simulink model "Rasmusson"  (Simulink 7.1)
settings: Solver=ode15s  StartTime=0.0  StopTime=500  FixedStep=1e-4  MaxStep=0.1  RelTol=1e-6
values from neighbouring files (symbols this model uses):
  Acap = 1.534e-4    (= 0.0001534)    [MMparameters.m]
  aKss = 0.417069e-3    (= 0.000417069)    [MMparameters.m]
  ato_f = 0.265563e-2    (= 0.00265563)    [MMparameters.m]
  ato_s = 0.417069e-3    (= 0.000417069)    [MMparameters.m]
  aur = 0.417069e-3    (= 0.000417069)    [MMparameters.m]
  C2 = 0.124216e-3    (= 0.000124216)    [MMparameters.m]
  C3 = 0.578679e-8    (= 5.78679e-09)    [MMparameters.m]
  C4 = 0.119816e-12    (= 1.19816e-13)    [MMparameters.m]
  Cai = 0.115001    [MMparameters.m]
  CaJSR = 1299.50    (= 1299.5)    [MMparameters.m]
  CaNSR = 1299.50    (= 1299.5)    [MMparameters.m]
  Cao = 1800    [MMparameters.m]
  Cass = 0.115001    [MMparameters.m]
  CK1 = 0.992513e-3    (= 0.000992513)    [MMparameters.m]
  CK2 = 0.641229e-3    (= 0.000641229)    [MMparameters.m]
  Cm = 1.0    (= 1)    [MMparameters.m]
  CMDN_tot = 50.0    (= 50)    [MMparameters.m]
  CNa1 = 0.279132e-3    (= 0.000279132)    [MMparameters.m]
  CNa2 = 0.020752    [MMparameters.m]
  CSQN_tot = 15000.0    (= 15000)    [MMparameters.m]
  ECa_L = 63.0    (= 63)    [MMparameters.m]
  ECl = -40.0    (= -40)    [MMparameters.m]
  F = 96.5    [MMparameters.m]
  GCab = 0.000367    [MMparameters.m]
  GCaL = 0.1729    [MMparameters.m]
  GCl_Ca = 10.0    (= 10)    [MMparameters.m]
  GKr = 0.078    [MMparameters.m]
  GKs = 0.00575    [MMparameters.m]
  GKss = 0.050    (= 0.05)    [MMparameters.m]
  GKtof = 0.4067    [MMparameters.m]
  GKtos = 0.0    (= 0)    [MMparameters.m]
  GKur = 0.160    (= 0.16)    [MMparameters.m]
  GNa = 13.0    (= 13)    [MMparameters.m]
  GNab = 0.0026    [MMparameters.m]
  HTRPN_tot = 140.0    (= 140)    [MMparameters.m]
  HTRPNCa = 125.290    (= 125.29)    [MMparameters.m]
  I1 = 0.497923e-18    (= 4.97923e-19)    [MMparameters.m]
  I1Na = 0.673345e-6    (= 6.73345e-07)    [MMparameters.m]
  I2 = 0.345847e-13    (= 3.45847e-14)    [MMparameters.m]
  I2Na = 0.155787e-8    (= 1.55787e-09)    [MMparameters.m]
  I3 = 0.185106e-13    (= 1.85106e-14)    [MMparameters.m]
  ICaL_max = 7.0    (= 7)    [MMparameters.m]
  ICNa2 = 0.0113879    [MMparameters.m]
  ICNa3 = 0.342780    (= 0.34278)    [MMparameters.m]
  IFNa = 0.153176e-3    (= 0.000153176)    [MMparameters.m]
  IK = 0.319129e-4    (= 3.19129e-05)    [MMparameters.m]
  iKss = 1.0    (= 1)    [MMparameters.m]
  INaK_max = 0.88    [MMparameters.m]
  Ip_Ca_max = 1.0    (= 1)    [MMparameters.m]
  ito_f = 0.999977    [MMparameters.m]
  ito_s = 0.998543    [MMparameters.m]
  iur = 0.998543    [MMparameters.m]
  ka1 = 0.006075    [MMparameters.m]
  ka2 = 0.07125    [MMparameters.m]
  kb = 0.036778    [MMparameters.m]
  kb1 = 0.00405    [MMparameters.m]
  kb2 = 0.965    [MMparameters.m]
  kc1 = 0.009    [MMparameters.m]
  kc2 = 0.0008    [MMparameters.m]
  kf = 0.023761    [MMparameters.m]
  khtrpn1 = 0.00237    [MMparameters.m]
  khtrpn2 = 3.2e-5    (= 3.2e-05)    [MMparameters.m]
  Ki = 143720    [MMparameters.m]
  kltrpn1 = 0.0327    [MMparameters.m]
  kltrpn2 = 0.0196    [MMparameters.m]
  Km_Ca = 1380    [MMparameters.m]
  Km_Cl = 10.0    (= 10)    [MMparameters.m]
  Km_CMDN = 0.238    [MMparameters.m]
  Km_CSQN = 800.0    (= 800)    [MMparameters.m]
  Km_Ko = 1500    [MMparameters.m]
  Km_Na = 87500    [MMparameters.m]
  Km_Nai = 21000    [MMparameters.m]
  Km_p_Ca = 0.5    [MMparameters.m]
  Km_up = 0.5    [MMparameters.m]
  kNaCa = 292.8    [MMparameters.m]
  Ko = 5400    [MMparameters.m]
  Kpc_half = 20.0    (= 20)    [MMparameters.m]
  Kpc_max = 0.23324    [MMparameters.m]
  Kpcb = 0.0005    [MMparameters.m]
  ksat = 0.1    [MMparameters.m]
  LTRPN_tot = 70.0    (= 70)    [MMparameters.m]
  LTRPNCa = 11.2684    [MMparameters.m]
  Nai = 14237.1    [MMparameters.m]
  Nao = 140000    [MMparameters.m]
  nKs = 0.262753e-3    (= 0.000262753)    [MMparameters.m]
  nu1 = 4.5    [MMparameters.m]
  nu2 = 1.74e-5    (= 1.74e-05)    [MMparameters.m]
  nu3 = 0.45    [MMparameters.m]
  O = 0.930308e-18    (= 9.30308e-19)    [MMparameters.m]
  OK = 0.175298e-3    (= 0.000175298)    [MMparameters.m]
  ONa = 0.713483e-6    (= 7.13483e-07)    [MMparameters.m]
  PC2 = 0.167740e-3    (= 0.00016774)    [MMparameters.m]
  PO1 = 0.149102e-4    (= 1.49102e-05)    [MMparameters.m]
  PO2 = 0.951726e-10    (= 9.51726e-11)    [MMparameters.m]
  PRyR = 0.0    (= 0)    [MMparameters.m]
  R = 8.314    [MMparameters.m]
  T = 298    [MMparameters.m]
  tautr = 20.0    (= 20)    [MMparameters.m]
  tauxfer = 8.0    (= 8)    [MMparameters.m]
  V = -82.4202    [MMparameters.m]
  VJSR = 0.12e-6    (= 1.2e-07)    [MMparameters.m]
  Vmyo = 25.84e-6    (= 2.584e-05)    [MMparameters.m]
  VNSR = 2.098e-6    (= 2.098e-06)    [MMparameters.m]
  Vss = 1.485e-9    (= 1.485e-09)    [MMparameters.m]
  yita = 0.35    [MMparameters.m]
(part 1 of 2)
settings Model: Creator=yunchen  LastModifiedBy=yunchen  BufferReuse=off
settings SolverCC: MaxOrder=2
settings DataIOCC: LimitDataPoints=off  SaveFinalState=on  SaveOutput=off  SignalLoggingName=sigsOut
settings OptimizationCC: InlineParams=on  OptimizeBlockIOStorage=off  BufferReuse=off  ExpressionFolding=off  LocalBlockOutputs=off
settings DebuggingCC: SaveWithParameterizedLinksMsg=none  MultiTaskDSMMsg=warning  MultiTaskCondExecSysMsg=none  CheckMatrixSingularityMsg=warning

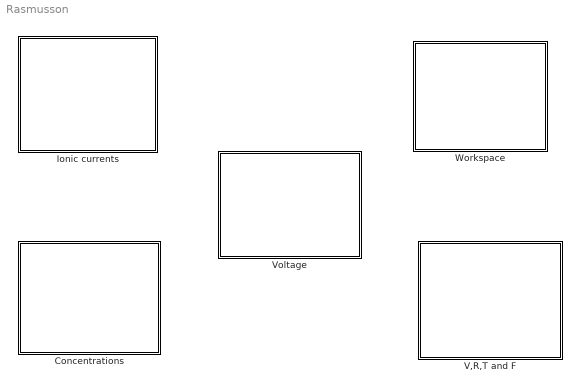
== system Rasmusson ==
  Concentrations : Subsystem
  Ionic currents : Subsystem
  V,R,T and F : Subsystem
  Voltage : Subsystem
  Workspace : Subsystem

== system Rasmusson/Concentrations ==
  ACdivideVF : Subsystem
  Caconcentration : Subsystem
  Ki : Subsystem
  Nai : Subsystem

== system Rasmusson/Ionic currents ==
  EK : Subsystem
  ENa : Subsystem
  ICaL : Subsystem
  ICab : Subsystem
  IK1 : Subsystem
  IKr : Subsystem
  IKs : Subsystem
  IKss : Subsystem
  IKto,f : Subsystem
  IKto,s : Subsystem
  IKur : Subsystem
  INa : Subsystem
  INaCa : Subsystem
  INaK : Subsystem
  INab : Subsystem
  IpCa : Subsystem

== system Rasmusson/V,R,T and F ==
  Divide : Product  Inputs=*/  OutDataType=sfix(16)  OutScaling=2^-10
  Divide1 : Product  Inputs=*/  OutDataType=sfix(16)  OutScaling=2^-10
  F : Constant  Value=F  OutDataType=sfix(16)  OutScaling=2^0
  Product : Product  OutDataType=sfix(16)  OutScaling=2^0  RndMeth=Zero
  R : Constant  Value=R  OutDataType=sfix(16)  OutScaling=2^0
  T : Constant  Value=T  OutDataType=sfix(16)  OutScaling=2^0
  tag scope: RTdivideF=global, VFdivideRT=global
  wires:
  R/1 -> Product/1
  T/1 -> Product/2
  Product/1 -> Divide/1
  F/1 -> Divide/2
  Divide/1 -> [RTdivideF], Divide1/2
  [volt] -> Divide1/1
  Divide1/1 -> [VFdivideRT]

== system Rasmusson/Voltage ==
  Cacurrents : Subsystem
  ICaCl : Subsystem
  Kdynamics : Subsystem
  Nadynamics : Subsystem
  Voltage : Subsystem

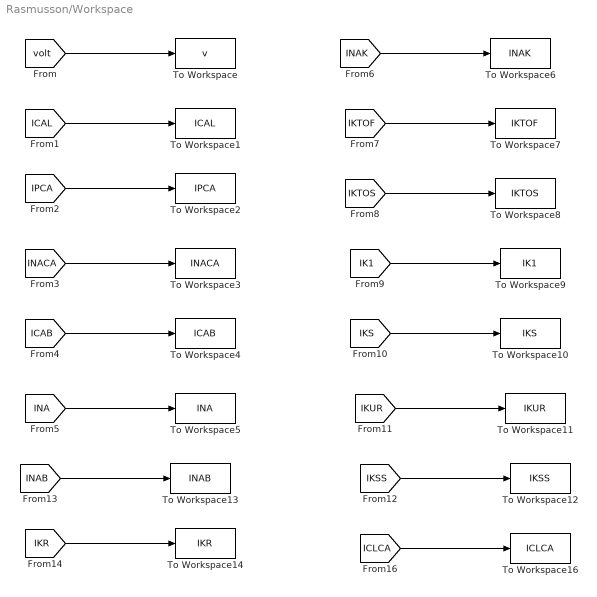
== system Rasmusson/Workspace ==
  To Workspace : ToWorkspace  VariableName=v  SampleTime=-1  SaveFormat=Array
  To Workspace1 : ToWorkspace  VariableName=ICAL  SampleTime=-1  SaveFormat=Array
  To Workspace10 : ToWorkspace  VariableName=IKS  SampleTime=-1  SaveFormat=Array
  To Workspace11 : ToWorkspace  VariableName=IKUR  SampleTime=-1  SaveFormat=Array
  To Workspace12 : ToWorkspace  VariableName=IKSS  SampleTime=-1  SaveFormat=Array
  To Workspace13 : ToWorkspace  VariableName=INAB  SampleTime=-1  SaveFormat=Array
  To Workspace14 : ToWorkspace  VariableName=IKR  SampleTime=-1  SaveFormat=Array
  To Workspace16 : ToWorkspace  VariableName=ICLCA  SampleTime=-1  SaveFormat=Array
  To Workspace2 : ToWorkspace  VariableName=IPCA  SampleTime=-1  SaveFormat=Array
  To Workspace3 : ToWorkspace  VariableName=INACA  SampleTime=-1  SaveFormat=Array
  To Workspace4 : ToWorkspace  VariableName=ICAB  SampleTime=-1  SaveFormat=Array
  To Workspace5 : ToWorkspace  VariableName=INA  SampleTime=-1  SaveFormat=Array
  To Workspace6 : ToWorkspace  VariableName=INAK  SampleTime=-1  SaveFormat=Array
  To Workspace7 : ToWorkspace  VariableName=IKTOF  SampleTime=-1  SaveFormat=Array
  To Workspace8 : ToWorkspace  VariableName=IKTOS  SampleTime=-1  SaveFormat=Array
  To Workspace9 : ToWorkspace  VariableName=IK1  SampleTime=-1  SaveFormat=Array
  wires:
  [volt] -> To Workspace/1
  [ICAL] -> To Workspace1/1
  [IPCA] -> To Workspace2/1
  [INACA] -> To Workspace3/1
  [ICAB] -> To Workspace4/1
  [INA] -> To Workspace5/1
  [INAK] -> To Workspace6/1
  [IKTOF] -> To Workspace7/1
  [IKTOS] -> To Workspace8/1
  [IK1] -> To Workspace9/1
  [IKS] -> To Workspace10/1
  [IKUR] -> To Workspace11/1
  [IKSS] -> To Workspace12/1
  [INAB] -> To Workspace13/1
  [IKR] -> To Workspace14/1
  [ICLCA] -> To Workspace16/1

== system Rasmusson/Concentrations/ACdivideVF ==
  Acap : Constant  Value=Acap  OutDataType=sfix(16)  OutScaling=2^0
  Cm : Constant  Value=Cm  OutDataType=sfix(16)  OutScaling=2^0
  Divide : Product  Inputs=**//  OutDataType=sfix(16)  OutScaling=2^-10
  F : Constant  Value=F  OutDataType=sfix(16)  OutScaling=2^0
  Vmyo : Constant  Value=Vmyo  OutDataType=sfix(16)  OutScaling=2^0
  tag scope: ACdivideVF=global
  wires:
  Acap/1 -> Divide/1
  Cm/1 -> Divide/2
  Vmyo/1 -> Divide/3
  F/1 -> Divide/4
  Divide/1 -> [ACdivideVF]

== system Rasmusson/Concentrations/Caconcentration ==
  Cabuffering : Subsystem
  Caconcentration : Subsystem
  Cafluxes : Subsystem
  Ryanodine_receptors : Subsystem

== system Rasmusson/Concentrations/Ki ==
  Add : Sum  Inputs=++++++++  OutDataType=sfix(16)  OutScaling=2^-10
  Gain : Gain  Gain=-1  ParameterDataType=sfix(16)  ParameterScaling=2^0  OutDataType=sfix(16)  OutScaling=2^0
  Gain1 : Gain  Gain=-2  ParameterDataType=sfix(16)  ParameterScaling=2^0  OutDataType=sfix(16)  OutScaling=2^0
  Integrator : Integrator  InitialConditionSource=external  InitialCondition=143720
  Ki : Constant  Value=Ki  OutDataType=sfix(16)  OutScaling=2^0
  Product : Product  OutDataType=sfix(16)  OutScaling=2^0  RndMeth=Zero
  tag scope: Ki=global
  wires:
  Integrator/1 -> [Ki]
  Gain/1 -> Integrator/1
  Product/1 -> Gain/1
  Add/1 -> Product/2
  [IKTOS] -> Add/2
  [IKTOF] -> Add/1
  [IK1] -> Add/3
  [IKS] -> Add/4
  [ACdivideVF] -> Product/1
  [IKSS] -> Add/5
  [IKUR] -> Add/6
  [IKR] -> Add/7
  Gain1/1 -> Add/8
  [INAK] -> Gain1/1
  Ki/1 -> Integrator/2

== system Rasmusson/Concentrations/Nai ==
  Add : Sum  Inputs=++++  OutDataType=sfix(16)  OutScaling=2^-10
  Gain : Gain  Gain=-1  ParameterDataType=sfix(16)  ParameterScaling=2^0  OutDataType=sfix(16)  OutScaling=2^0
  Gain1 : Gain  Gain=3  ParameterDataType=sfix(16)  ParameterScaling=2^0  OutDataType=sfix(16)  OutScaling=2^0
  Gain2 : Gain  Gain=3  ParameterDataType=sfix(16)  ParameterScaling=2^0  OutDataType=sfix(16)  OutScaling=2^0
  Integrator : Integrator  InitialConditionSource=external  InitialCondition=14237.1
  Nai : Constant  Value=Nai  OutDataType=sfix(16)  OutScaling=2^0
  Product : Product  OutDataType=sfix(16)  OutScaling=2^0  RndMeth=Zero
  tag scope: Nai=global
  wires:
  Integrator/1 -> [Nai]
  Gain/1 -> Integrator/1
  Product/1 -> Gain/1
  Add/1 -> Product/2
  Gain1/1 -> Add/4
  Gain2/1 -> Add/3
  [INAB] -> Add/2
  [INA] -> Add/1
  [INACA] -> Gain2/1
  [INAK] -> Gain1/1
  [ACdivideVF] -> Product/1
  Nai/1 -> Integrator/2

== system Rasmusson/Ionic currents/EK ==
  Divide : Product  Inputs=*/  OutDataType=sfix(16)  OutScaling=2^-10
  Ko : Constant  Value=Ko  OutDataType=sfix(16)  OutScaling=2^0
  Math Function : Math  Operator=log  OutDataType=sfix(16)  OutScaling=2^0  SaturateOnIntegerOverflow=on
  Product : Product  OutDataType=sfix(16)  OutScaling=2^0  RndMeth=Zero
  tag scope: EK=global
  wires:
  Ko/1 -> Divide/1
  [Ki] -> Divide/2
  Divide/1 -> Math Function/1
  Product/1 -> [EK]
  Math Function/1 -> Product/2
  [RTdivideF] -> Product/1

== system Rasmusson/Ionic currents/ENa ==
  Add : Sum  OutDataType=sfix(16)  OutScaling=2^-10
  Add1 : Sum  OutDataType=sfix(16)  OutScaling=2^-10
  Divide : Product  Inputs=*/  OutDataType=sfix(16)  OutScaling=2^-10
  Divide1 : Product  Inputs=**  OutDataType=sfix(16)  OutScaling=2^-10
  Gain : Gain  Gain=0.9  ParameterDataType=sfix(16)  ParameterScaling=2^0  OutDataType=sfix(16)  OutScaling=2^0
  Gain1 : Gain  Gain=0.1  ParameterDataType=sfix(16)  ParameterScaling=2^0  OutDataType=sfix(16)  OutScaling=2^0
  Gain2 : Gain  Gain=0.9  ParameterDataType=sfix(16)  ParameterScaling=2^0  OutDataType=sfix(16)  OutScaling=2^0
  Gain3 : Gain  Gain=0.1  ParameterDataType=sfix(16)  ParameterScaling=2^0  OutDataType=sfix(16)  OutScaling=2^0
  Ko : Constant  Value=Ko  OutDataType=sfix(16)  OutScaling=2^0
  Math Function : Math  Operator=log  OutDataType=sfix(16)  OutScaling=2^0  SaturateOnIntegerOverflow=on
  Nao : Constant  Value=Nao  OutDataType=sfix(16)  OutScaling=2^0
  tag scope: ENa=global
  wires:
  Divide/1 -> Math Function/1
  Gain/1 -> Add/1
  Add/1 -> Divide/1
  Gain1/1 -> Add/2
  Add1/1 -> Divide/2
  Gain2/1 -> Add1/1
  Gain3/1 -> Add1/2
  Math Function/1 -> Divide1/1
  [RTdivideF] -> Divide1/2
  Divide1/1 -> [ENa]
  [Ki] -> Gain3/1
  [Nai] -> Gain2/1
  Nao/1 -> Gain/1
  Ko/1 -> Gain1/1

== system Rasmusson/Ionic currents/ICaL ==
  ECaL : Constant  Value=ECa_L  OutDataType=sfix(16)  OutScaling=2^0
  GCaL : Constant  Value=GCaL  OutDataType=sfix(16)  OutScaling=2^0
  O : Subsystem
  Product : Product  Inputs=3  OutDataType=sfix(16)  OutScaling=2^0  RndMeth=Zero
  Subtract : Sum  Inputs=+-  OutDataType=sfix(16)  OutScaling=2^-10
  tag scope: ICAL=global
  wires:
  Product/1 -> [ICAL]
  [O] -> Product/2
  Subtract/1 -> Product/3
  [volt] -> Subtract/1
  GCaL/1 -> Product/1
  ECaL/1 -> Subtract/2

== system Rasmusson/Ionic currents/ICab ==
  ECaN : Subsystem
  GCab : Constant  Value=GCab  OutDataType=sfix(16)  OutScaling=2^0
  Product : Product  OutDataType=sfix(16)  OutScaling=2^0  RndMeth=Zero
  Subtract : Sum  Inputs=+-  OutDataType=sfix(16)  OutScaling=2^-10
  tag scope: ICAB=global
  wires:
  Product/1 -> [ICAB]
  [volt] -> Subtract/1
  [ECaN] -> Subtract/2
  Subtract/1 -> Product/2
  GCab/1 -> Product/1

== system Rasmusson/Ionic currents/IK1 ==
  Add : Sum  OutDataType=sfix(16)  OutScaling=2^-10
  Add1 : Sum  OutDataType=sfix(16)  OutScaling=2^-10
  Constant1 : Constant  Value=210  OutDataType=sfix(16)  OutScaling=2^0
  Constant2 : Constant  OutDataType=sfix(16)  OutScaling=2^0
  Divide : Product  Inputs=*/  OutDataType=sfix(16)  OutScaling=2^-10
  Divide1 : Product  Inputs=*/  OutDataType=sfix(16)  OutScaling=2^-10
  Gain : Gain  Gain=0.2938  ParameterDataType=sfix(16)  ParameterScaling=2^0  OutDataType=sfix(16)  OutScaling=2^0
  Gain1 : Gain  Gain=0.0896  ParameterDataType=sfix(16)  ParameterScaling=2^0  OutDataType=sfix(16)  OutScaling=2^0
  Ko : Constant  Value=Ko  OutDataType=sfix(16)  OutScaling=2^0
  Math Function : Math  OutDataType=sfix(16)  OutScaling=2^0  SaturateOnIntegerOverflow=on
  Product : Product  OutDataType=sfix(16)  OutScaling=2^0  RndMeth=Zero
  Subtract : Sum  Inputs=+-  OutDataType=sfix(16)  OutScaling=2^-10
  tag scope: IK1=global
  wires:
  Product/1 -> Gain/1
  Gain/1 -> [IK1]
  Divide/1 -> Product/1
  Ko/1 -> Divide/1, Add/1
  Add/1 -> Divide/2
  Constant1/1 -> Add/2
  [volt] -> Subtract/1
  [EK] -> Subtract/2
  Divide1/1 -> Product/2
  Subtract/1 -> Divide1/1, Gain1/1
  Add1/1 -> Divide1/2
  Constant2/1 -> Add1/2
  Math Function/1 -> Add1/1
  Gain1/1 -> Math Function/1

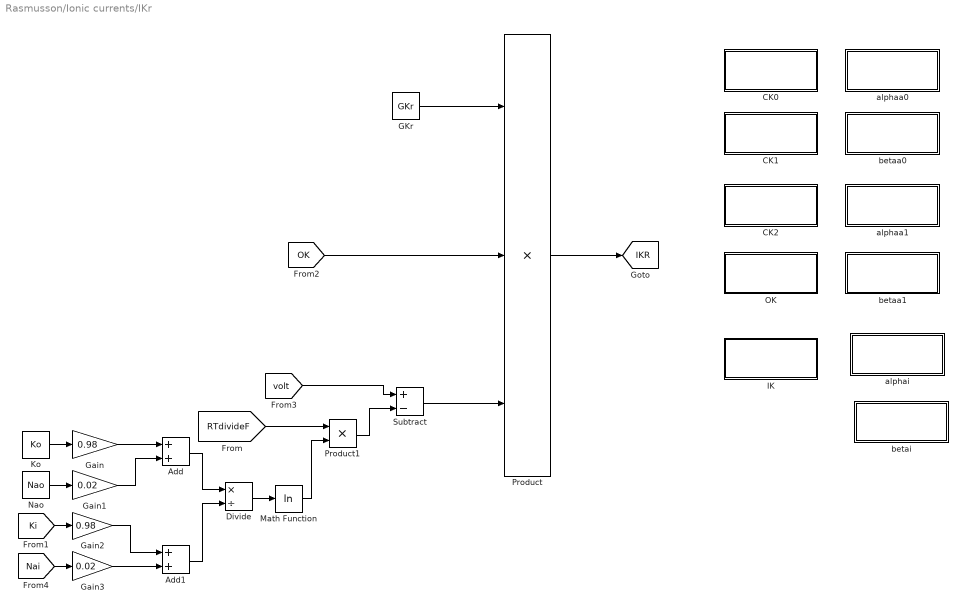
== system Rasmusson/Ionic currents/IKr ==
  Add : Sum  OutDataType=sfix(16)  OutScaling=2^-10
  Add1 : Sum  OutDataType=sfix(16)  OutScaling=2^-10
  CK0 : Subsystem
  CK1 : Subsystem
  CK2 : Subsystem
  Divide : Product  Inputs=*/  OutDataType=sfix(16)  OutScaling=2^-10
  GKr : Constant  Value=GKr  OutDataType=sfix(16)  OutScaling=2^0
  Gain : Gain  Gain=0.98  ParameterDataType=sfix(16)  ParameterScaling=2^0  OutDataType=sfix(16)  OutScaling=2^0
  Gain1 : Gain  Gain=0.02  ParameterDataType=sfix(16)  ParameterScaling=2^0  OutDataType=sfix(16)  OutScaling=2^0
  Gain2 : Gain  Gain=0.98  ParameterDataType=sfix(16)  ParameterScaling=2^0  OutDataType=sfix(16)  OutScaling=2^0
  Gain3 : Gain  Gain=0.02  ParameterDataType=sfix(16)  ParameterScaling=2^0  OutDataType=sfix(16)  OutScaling=2^0
  IK : Subsystem
  Ko : Constant  Value=Ko  OutDataType=sfix(16)  OutScaling=2^0
  Math Function : Math  Operator=log  OutDataType=sfix(16)  OutScaling=2^0  SaturateOnIntegerOverflow=on
  Nao : Constant  Value=Nao  OutDataType=sfix(16)  OutScaling=2^0
  OK : Subsystem
  Product : Product  Inputs=3  OutDataType=sfix(16)  OutScaling=2^0  RndMeth=Zero
  Product1 : Product  OutDataType=sfix(16)  OutScaling=2^0  RndMeth=Zero
  Subtract : Sum  Inputs=+-  OutDataType=sfix(16)  OutScaling=2^-10
  alphaa0 : Subsystem
  alphaa1 : Subsystem
  alphai : Subsystem
  betaa0 : Subsystem
  betaa1 : Subsystem
  betai : Subsystem
  tag scope: IKR=global
  wires:
  Product/1 -> [IKR]
  GKr/1 -> Product/1
  [OK] -> Product/2
  Subtract/1 -> Product/3
  [volt] -> Subtract/1
  Product1/1 -> Subtract/2
  [RTdivideF] -> Product1/1
  Math Function/1 -> Product1/2
  Divide/1 -> Math Function/1
  Add/1 -> Divide/1
  Add1/1 -> Divide/2
  Gain/1 -> Add/1
  Ko/1 -> Gain/1
  Gain1/1 -> Add/2
  Nao/1 -> Gain1/1
  [Ki] -> Gain2/1
  [Nai] -> Gain3/1
  Gain2/1 -> Add1/1
  Gain3/1 -> Add1/2

== system Rasmusson/Ionic currents/IKs ==
  Divide : Product  Inputs=***  OutDataType=sfix(16)  OutScaling=2^-10
  GKs : Constant  Value=GKs  OutDataType=sfix(16)  OutScaling=2^0
  Product : Product  OutDataType=sfix(16)  OutScaling=2^0  RndMeth=Zero
  Subtract : Sum  Inputs=+-  OutDataType=sfix(16)  OutScaling=2^-10
  alphan : Subsystem
  betan : Subsystem
  nKs : Subsystem
  tag scope: IKS=global
  wires:
  GKs/1 -> Divide/1
  Product/1 -> Divide/2
  Subtract/1 -> Divide/3
  Divide/1 -> [IKS]
  [EK] -> Subtract/2
  [volt] -> Subtract/1
  [nKs] -> Product/1, Product/2

== system Rasmusson/Ionic currents/IKss ==
  GKss : Constant  Value=GKss  OutDataType=sfix(16)  OutScaling=2^0
  Product : Product  Inputs=4  OutDataType=sfix(16)  OutScaling=2^0  RndMeth=Zero
  Subtract : Sum  Inputs=+-  OutDataType=sfix(16)  OutScaling=2^-10
  aKss : Subsystem
  iKss : Subsystem
  tauKss : Subsystem
  tag scope: IKSS=global
  wires:
  [EK] -> Subtract/2
  [volt] -> Subtract/1
  Subtract/1 -> Product/4
  Product/1 -> [IKSS]
  GKss/1 -> Product/1
  [aKss] -> Product/2
  [iKss] -> Product/3

== system Rasmusson/Ionic currents/IKto,f ==
  Divide : Product  Inputs=****  OutDataType=sfix(16)  OutScaling=2^-10
  GKtof : Constant  Value=GKtof  OutDataType=sfix(16)  OutScaling=2^0
  Product : Product  Inputs=3  OutDataType=sfix(16)  OutScaling=2^0  RndMeth=Zero
  Subtract : Sum  Inputs=+-  OutDataType=sfix(16)  OutScaling=2^-10
  alphaa : Subsystem
  alphaj : Subsystem
  atof : Subsystem
  betaa : Subsystem
  betaj : Subsystem
  itof : Subsystem
  tag scope: IKTOF=global
  wires:
  [volt] -> Subtract/1
  [EK] -> Subtract/2
  Divide/1 -> [IKTOF]
  Subtract/1 -> Divide/4
  [atof] -> Product/1, Product/2, Product/3
  Product/1 -> Divide/2
  [itof] -> Divide/3
  GKtof/1 -> Divide/1

== system Rasmusson/Ionic currents/IKto,s ==
  GKtos : Constant  Value=GKtos  OutDataType=sfix(16)  OutScaling=2^0
  Product : Product  Inputs=4  OutDataType=sfix(16)  OutScaling=2^0  RndMeth=Zero
  Subtract : Sum  Inputs=+-  OutDataType=sfix(16)  OutScaling=2^-10
  ass : Subsystem
  atos : Subsystem
  iss : Subsystem
  itos : Subsystem
  tautas : Subsystem
  tautis : Subsystem
  tag scope: IKTOS=global
  wires:
  [EK] -> Subtract/2
  [volt] -> Subtract/1
  Subtract/1 -> Product/4
  Product/1 -> [IKTOS]
  GKtos/1 -> Product/1
  [atos] -> Product/2
  [itos] -> Product/3

== system Rasmusson/Ionic currents/IKur ==
  GKur : Constant  Value=GKur  OutDataType=sfix(16)  OutScaling=2^0
  Product : Product  Inputs=4  OutDataType=sfix(16)  OutScaling=2^0  RndMeth=Zero
  Subtract : Sum  Inputs=+-  OutDataType=sfix(16)  OutScaling=2^-10
  aur : Subsystem
  iur : Subsystem
  tauaur : Subsystem
  tauiur : Subsystem
  tag scope: IKUR=global
  wires:
  [iur] -> Product/3
  [aur] -> Product/2
  GKur/1 -> Product/1
  Product/1 -> [IKUR]
  Subtract/1 -> Product/4
  [volt] -> Subtract/1
  [EK] -> Subtract/2

== system Rasmusson/Ionic currents/INa ==
  GNa : Constant  Value=GNa  OutDataType=sfix(16)  OutScaling=2^0
  ONa : Subsystem
  Product : Product  Inputs=3  OutDataType=sfix(16)  OutScaling=2^0  RndMeth=Zero
  Subtract : Sum  Inputs=+-  OutDataType=sfix(16)  OutScaling=2^-10
  tag scope: INA=global
  wires:
  Product/1 -> [INA]
  [ONa] -> Product/2
  Subtract/1 -> Product/3
  [volt] -> Subtract/1
  GNa/1 -> Product/1
  [ENa] -> Subtract/2

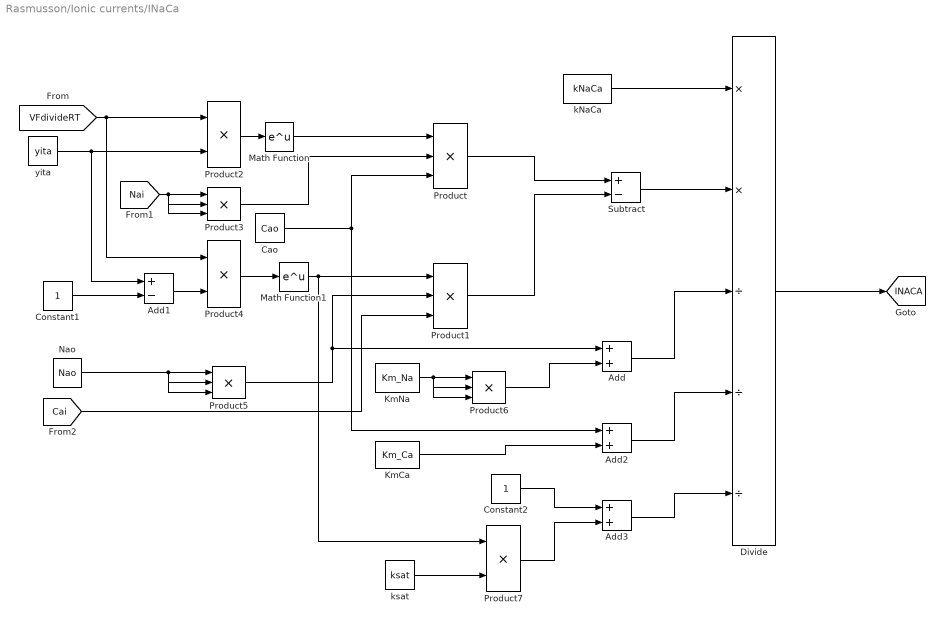
== system Rasmusson/Ionic currents/INaCa ==
  Add : Sum  OutDataType=sfix(16)  OutScaling=2^-10
  Add1 : Sum  Inputs=+-  OutDataType=sfix(16)  OutScaling=2^-10
  Add2 : Sum  OutDataType=sfix(16)  OutScaling=2^-10
  Add3 : Sum  OutDataType=sfix(16)  OutScaling=2^-10
  Cao : Constant  Value=Cao  OutDataType=sfix(16)  OutScaling=2^0
  Constant1 : Constant  OutDataType=sfix(16)  OutScaling=2^0
  Constant2 : Constant  OutDataType=sfix(16)  OutScaling=2^0
  Divide : Product  Inputs=**///  OutDataType=sfix(16)  OutScaling=2^-10
  KmCa : Constant  Value=Km_Ca  OutDataType=sfix(16)  OutScaling=2^0
  KmNa : Constant  Value=Km_Na  OutDataType=sfix(16)  OutScaling=2^0
  Math Function : Math  OutDataType=sfix(16)  OutScaling=2^0  SaturateOnIntegerOverflow=on
  Math Function1 : Math  OutDataType=sfix(16)  OutScaling=2^0  SaturateOnIntegerOverflow=on
  Nao : Constant  Value=Nao  OutDataType=sfix(16)  OutScaling=2^0
  Product{,1,3,5..6} (5 alike) : Product  Inputs=3  OutDataType=sfix(16)  OutScaling=2^0  RndMeth=Zero
  Product2 : Product  OutDataType=sfix(16)  OutScaling=2^0  RndMeth=Zero
  Product4 : Product  OutDataType=sfix(16)  OutScaling=2^0  RndMeth=Zero
  Product7 : Product  OutDataType=sfix(16)  OutScaling=2^0  RndMeth=Zero
  Subtract : Sum  Inputs=+-  OutDataType=sfix(16)  OutScaling=2^-10
  kNaCa : Constant  Value=kNaCa  OutDataType=sfix(16)  OutScaling=2^0
  ksat : Constant  Value=ksat  OutDataType=sfix(16)  OutScaling=2^0
  yita : Constant  Value=yita  OutDataType=sfix(16)  OutScaling=2^0
  tag scope: INACA=global
  wires:
  Divide/1 -> [INACA]
  kNaCa/1 -> Divide/1
  Subtract/1 -> Divide/2
  Product/1 -> Subtract/1
  Product1/1 -> Subtract/2
  Math Function/1 -> Product/1
  Product2/1 -> Math Function/1
  yita/1 -> Product2/2, Add1/1
  [Nai] -> Product3/1, Product3/2, Product3/3
  Product3/1 -> Product/2
  Cao/1 -> Product/3, Add2/1
  Math Function1/1 -> Product1/1, Product7/1
  Product4/1 -> Math Function1/1
  Add1/1 -> Product4/2
  Constant1/1 -> Add1/2
  Nao/1 -> Product5/1, Product5/2, Product5/3
  Product5/1 -> Product1/2, Add/1
  [Cai] -> Product1/3
  Add/1 -> Divide/3
  Product6/1 -> Add/2
  KmNa/1 -> Product6/1, Product6/2, Product6/3
  Add2/1 -> Divide/4
  KmCa/1 -> Add2/2
  Add3/1 -> Divide/5
  Constant2/1 -> Add3/1
  Product7/1 -> Add3/2
  ksat/1 -> Product7/2
  [VFdivideRT] -> Product2/1, Product4/1

== system Rasmusson/Ionic currents/INaK ==
  Add : Sum  OutDataType=sfix(16)  OutScaling=2^-10
  Add1 : Sum  OutDataType=sfix(16)  OutScaling=2^-10
  Constant2 : Constant  OutDataType=sfix(16)  OutScaling=2^0
  Divide : Product  Inputs=***//  OutDataType=sfix(16)  OutScaling=2^-10
  Divide1 : Product  Inputs=*/  OutDataType=sfix(16)  OutScaling=2^-10
  Fcn : Fcn  Expr=sqrt(u*u*u)
  INaKmax : Constant  Value=INaK_max  OutDataType=sfix(16)  OutScaling=2^0
  KmK0 : Constant  Value=Km_Ko  OutDataType=sfix(16)  OutScaling=2^0
  KmNai : Constant  Value=Km_Nai  OutDataType=sfix(16)  OutScaling=2^0
  Ko : Constant  Value=Ko  OutDataType=sfix(16)  OutScaling=2^0
  fNaK : Subsystem
  tag scope: INAK=global
  wires:
  Divide/1 -> [INAK]
  INaKmax/1 -> Divide/1
  [fNaK] -> Divide/2
  Ko/1 -> Divide/3, Add1/1
  Constant2/1 -> Add/1
  Fcn/1 -> Add/2
  Divide1/1 -> Fcn/1
  [Nai] -> Divide1/2
  KmNai/1 -> Divide1/1
  Add/1 -> Divide/5
  Add1/1 -> Divide/4
  KmK0/1 -> Add1/2

== system Rasmusson/Ionic currents/INab ==
  GNab : Constant  Value=GNab  OutDataType=sfix(16)  OutScaling=2^0
  Product : Product  OutDataType=sfix(16)  OutScaling=2^0  RndMeth=Zero
  Subtract : Sum  Inputs=+-  OutDataType=sfix(16)  OutScaling=2^-10
  tag scope: INAB=global
  wires:
  Product/1 -> [INAB]
  GNab/1 -> Product/1
  Subtract/1 -> Product/2
  [volt] -> Subtract/1
  [ENa] -> Subtract/2

== system Rasmusson/Ionic currents/IpCa ==
  Add : Sum  OutDataType=sfix(16)  OutScaling=2^-10
  Divide : Product  Inputs=**/  OutDataType=sfix(16)  OutScaling=2^-10
  IpCamax : Constant  Value=Ip_Ca_max  OutDataType=sfix(16)  OutScaling=2^0
  KmpCa : Constant  Value=Km_p_Ca  OutDataType=sfix(16)  OutScaling=2^0
  square : Product  Inputs=**  OutDataType=sfix(16)  OutScaling=2^-10
  square1 : Product  Inputs=**  OutDataType=sfix(16)  OutScaling=2^-10
  tag scope: IPCA=global
  wires:
  Divide/1 -> [IPCA]
  IpCamax/1 -> Divide/1
  [Cai] -> square1/1, square1/2
  square1/1 -> Divide/2, Add/1
  Add/1 -> Divide/3
  square/1 -> Add/2
  KmpCa/1 -> square/1, square/2

== system Rasmusson/Voltage/Cacurrents ==
  Add : Sum  Inputs=++++  OutDataType=sfix(16)  OutScaling=2^-10
  tag scope: Cacurrents=global
  wires:
  Add/1 -> [Cacurrents]
  [ICAL] -> Add/1
  [IPCA] -> Add/2
  [INACA] -> Add/3
  [ICAB] -> Add/4

== system Rasmusson/Voltage/ICaCl ==
  Add : Sum  OutDataType=sfix(16)  OutScaling=2^-10
  Divide : Product  Inputs=****/  OutDataType=sfix(16)  OutScaling=2^-10
  ECl : Constant  Value=ECl  OutDataType=sfix(16)  OutScaling=2^0
  GClCa : Constant  Value=GCl_Ca  OutDataType=sfix(16)  OutScaling=2^0
  KmCl : Constant  Value=Km_Cl  OutDataType=sfix(16)  OutScaling=2^0
  OClCa : Subsystem
  Subtract : Sum  Inputs=+-  OutDataType=sfix(16)  OutScaling=2^-10
  tag scope: ICLCA=global
  wires:
  Divide/1 -> [ICLCA]
  GClCa/1 -> Divide/1
  [OClCa] -> Divide/2
  [volt] -> Subtract/1
  ECl/1 -> Subtract/2
  KmCl/1 -> Add/2
  Add/1 -> Divide/5
  [Cai] -> Divide/4, Add/1
  Subtract/1 -> Divide/3

== system Rasmusson/Voltage/Kdynamics ==
  Add : Sum  Inputs=++++++++  OutDataType=sfix(16)  OutScaling=2^-10
  tag scope: Kdynamics=global
  wires:
  Add/1 -> [Kdynamics]
  [IKTOF] -> Add/1
  [IKTOS] -> Add/2
  [IK1] -> Add/3
  [IKS] -> Add/4
  [IKUR] -> Add/5
  [IKSS] -> Add/6
  [IKR] -> Add/7
  [INAK] -> Add/8

== system Rasmusson/Voltage/Nadynamics ==
  Add : Sum  OutDataType=sfix(16)  OutScaling=2^-10
  tag scope: Nadynamics=global
  wires:
  Add/1 -> [Nadynamics]
  [INA] -> Add/1
  [INAB] -> Add/2

== system Rasmusson/Voltage/Voltage ==
  Add : Sum  Inputs=+++++  OutDataType=sfix(16)  OutScaling=2^-10
  Cm : Constant  Value=Cm  OutDataType=sfix(16)  OutScaling=2^0
  Divide : Product  Inputs=*/  OutDataType=sfix(16)  OutScaling=2^-10
  From Workspace : FromWorkspace  VariableName=I_ext  SampleTime=0
  Gain : Gain  Gain=-1  ParameterDataType=sfix(16)  ParameterScaling=2^0  OutDataType=sfix(16)  OutScaling=2^0
  Integrator : Integrator  InitialConditionSource=external  InitialCondition=-82.4202
  Scope : Scope
      settings: YMin=-83  YMax=-78.25
  V : Constant  Value=V  OutDataType=sfix(16)  OutScaling=2^0
  tag scope: volt=global
  wires:
  Integrator/1 -> [volt], Scope/1
  Divide/1 -> Integrator/1
  Add/1 -> Divide/1
  [Cacurrents] -> Add/1
  [Nadynamics] -> Add/2
  [Kdynamics] -> Add/3
  [ICLCA] -> Add/4
  From Workspace/1 -> Add/5
  Gain/1 -> Divide/2
  Cm/1 -> Gain/1
  V/1 -> Integrator/2

== system Rasmusson/Concentrations/Caconcentration/Cabuffering ==
  HTRPNCa : Subsystem
  LTRPNCa : Subsystem

== system Rasmusson/Concentrations/Caconcentration/Caconcentration ==
  BJSR : Subsystem
  Bi : Subsystem
  Bss : Subsystem
  CaJSR : Subsystem
  CaNSR : Subsystem
  Cai : Subsystem
  Cass : Subsystem

== system Rasmusson/Concentrations/Caconcentration/Cafluxes ==
  Jleak : Subsystem
  Jrel : Subsystem
  Jtr : Subsystem
  Jtrpn : Subsystem
  Jup : Subsystem
  Jxfer : Subsystem
  PRyR : Subsystem

== system Rasmusson/Concentrations/Caconcentration/Ryanodine_receptors ==
  PC1 : Subsystem
  PC2 : Subsystem
  PO1 : Subsystem
  PO2 : Subsystem

== system Rasmusson/Ionic currents/ICaL/O ==
  C1 : Subsystem
  C2 : Subsystem
  C3 : Subsystem
  C4 : Subsystem
  I1 : Subsystem
  I2 : Subsystem
  I3 : Subsystem
  Kpcb : Subsystem
  Kpcf : Subsystem
  O1 : Subsystem
  alpha : Subsystem
  beta : Subsystem
  gamma : Subsystem

== system Rasmusson/Ionic currents/ICab/ECaN ==
  Cao : Constant  Value=Cao  OutDataType=sfix(16)  OutScaling=2^0
  Divide : Product  Inputs=*/  OutDataType=sfix(16)  OutScaling=2^-10
  Divide1 : Product  Inputs=**  OutDataType=sfix(16)  OutScaling=2^-10
  Gain : Gain  Gain=0.5  ParameterDataType=sfix(16)  ParameterScaling=2^0  OutDataType=sfix(16)  OutScaling=2^0
  Math Function : Math  Operator=log  OutDataType=sfix(16)  OutScaling=2^0  SaturateOnIntegerOverflow=on
  tag scope: ECaN=global
  wires:
  [RTdivideF] -> Gain/1
  Cao/1 -> Divide/1
  [Cai] -> Divide/2
  Divide/1 -> Math Function/1
  Math Function/1 -> Divide1/1
  Gain/1 -> Divide1/2
  Divide1/1 -> [ECaN]

== system Rasmusson/Ionic currents/IKr/CK0 ==
  Add : Sum  Inputs=+----  OutDataType=sfix(16)  OutScaling=2^-10
  Constant : Constant  OutDataType=sfix(16)  OutScaling=2^0
  tag scope: CK0=global
  wires:
  Add/1 -> [CK0]
  Constant/1 -> Add/1
  [CK1] -> Add/2
  [CK2] -> Add/3
  [OK] -> Add/4
  [IK] -> Add/5

== system Rasmusson/Ionic currents/IKr/CK1 ==
  Add : Sum  Inputs=++--  OutDataType=sfix(16)  OutScaling=2^-10
  CK1 : Constant  Value=CK1  OutDataType=sfix(16)  OutScaling=2^0
  Integrator : Integrator  InitialConditionSource=external  InitialCondition=0.992513e-3
  Product{,1..3} (4 alike) : Product  OutDataType=sfix(16)  OutScaling=2^0  RndMeth=Zero
  kb : Constant  Value=kb  OutDataType=sfix(16)  OutScaling=2^0
  kf : Constant  Value=kf  OutDataType=sfix(16)  OutScaling=2^0
  tag scope: CK1=global
  wires:
  Add/1 -> Integrator/1
  Integrator/1 -> [CK1], Product2/2, Product3/2
  Product/1 -> Add/1
  Product1/1 -> Add/2
  Product2/1 -> Add/3
  Product3/1 -> Add/4
  kf/1 -> Product3/1
  [betaa0] -> Product2/1
  kb/1 -> Product1/1
  [CK2] -> Product1/2
  [CK0] -> Product/2
  [alphaa0] -> Product/1
  CK1/1 -> Integrator/2

== system Rasmusson/Ionic currents/IKr/CK2 ==
  Add : Sum  Inputs=++--  OutDataType=sfix(16)  OutScaling=2^-10
  CK2 : Constant  Value=CK2  OutDataType=sfix(16)  OutScaling=2^0
  Integrator : Integrator  InitialConditionSource=external  InitialCondition=0.641229e-3
  Product{,1..3} (4 alike) : Product  OutDataType=sfix(16)  OutScaling=2^0  RndMeth=Zero
  kb : Constant  Value=kb  OutDataType=sfix(16)  OutScaling=2^0
  kf : Constant  Value=kf  OutDataType=sfix(16)  OutScaling=2^0
  tag scope: CK2=global
  wires:
  [betaa1] -> Product/1
  [OK] -> Product/2
  [CK1] -> Product1/2
  kf/1 -> Product1/1
  [alphaa1] -> Product2/1
  kb/1 -> Product3/1
  Product3/1 -> Add/4
  Product2/1 -> Add/3
  Product1/1 -> Add/2
  Product/1 -> Add/1
  Integrator/1 -> Product3/2, Product2/2, [CK2]
  Add/1 -> Integrator/1
  CK2/1 -> Integrator/2

== system Rasmusson/Ionic currents/IKr/IK ==
  IK : Constant  Value=IK  OutDataType=sfix(16)  OutScaling=2^0
  Integrator : Integrator  InitialConditionSource=external  InitialCondition=0.319129e-4
  Product : Product  OutDataType=sfix(16)  OutScaling=2^0  RndMeth=Zero
  Product1 : Product  OutDataType=sfix(16)  OutScaling=2^0  RndMeth=Zero
  Subtract : Sum  Inputs=+-  OutDataType=sfix(16)  OutScaling=2^-10
  tag scope: IK=global
  wires:
  Subtract/1 -> Integrator/1
  Integrator/1 -> [IK], Product1/2
  Product/1 -> Subtract/1
  Product1/1 -> Subtract/2
  [alphai] -> Product/1
  [OK] -> Product/2
  [betai] -> Product1/1
  IK/1 -> Integrator/2

== system Rasmusson/Ionic currents/IKr/OK ==
  Add : Sum  Inputs=++--  OutDataType=sfix(16)  OutScaling=2^-10
  Integrator : Integrator  InitialConditionSource=external  InitialCondition=0.175298e-3
  OK : Constant  Value=OK  OutDataType=sfix(16)  OutScaling=2^0
  Product{,1..3} (4 alike) : Product  OutDataType=sfix(16)  OutScaling=2^0  RndMeth=Zero
  tag scope: OK=global
  wires:
  Add/1 -> Integrator/1
  Integrator/1 -> [OK], Product2/2, Product3/2
  Product/1 -> Add/1
  Product1/1 -> Add/2
  Product2/1 -> Add/3
  Product3/1 -> Add/4
  [alphai] -> Product3/1
  [betaa1] -> Product2/1
  [betai] -> Product1/1
  [IK] -> Product1/2
  [CK2] -> Product/2
  [alphaa1] -> Product/1
  OK/1 -> Integrator/2

== system Rasmusson/Ionic currents/IKr/alphaa0 ==
  alphaa0 : Fcn  Expr=0.022348*exp(0.01176*u)
  tag scope: alphaa0=global
  wires:
  [volt] -> alphaa0/1
  alphaa0/1 -> [alphaa0]

== system Rasmusson/Ionic currents/IKr/alphaa1 ==
  alphaa1 : Fcn  Expr=0.013733*exp(0.038198*u)
  tag scope: alphaa1=global
  wires:
  [volt] -> alphaa1/1
  alphaa1/1 -> [alphaa1]

== system Rasmusson/Ionic currents/IKr/alphai ==
  alphai : Fcn  Expr=0.090821*exp(0.023391*(u+5))
  tag scope: alphai=global
  wires:
  [volt] -> alphai/1
  alphai/1 -> [alphai]

== system Rasmusson/Ionic currents/IKr/betaa0 ==
  betaa0 : Fcn  Expr=0.047002*exp(-0.0631*u)
  tag scope: betaa0=global
  wires:
  betaa0/1 -> [betaa0]
  [volt] -> betaa0/1

== system Rasmusson/Ionic currents/IKr/betaa1 ==
  betaa1 : Fcn  Expr=0.0000689*exp(-0.04178*u)
  tag scope: betaa1=global
  wires:
  betaa1/1 -> [betaa1]
  [volt] -> betaa1/1

== system Rasmusson/Ionic currents/IKr/betai ==
  betai : Fcn  Expr=0.006497*exp(-0.03268*(u+5))
  tag scope: betai=global
  wires:
  betai/1 -> [betai]
  [volt] -> betai/1

== system Rasmusson/Ionic currents/IKs/alphan ==
  alphan : Fcn  Expr=0.00000481333*(u+26.5)/(1-exp(-0.128*(u+26.5)))
  tag scope: alphan=global
  wires:
  [volt] -> alphan/1
  alphan/1 -> [alphan]

== system Rasmusson/Ionic currents/IKs/betan ==
  betan : Fcn  Expr=0.0000953333*exp(-0.038*(u+26.5))
  tag scope: betan=global
  wires:
  betan/1 -> [betan]
  [volt] -> betan/1

== system Rasmusson/Ionic currents/IKs/nKs ==
  Constant : Constant  OutDataType=sfix(16)  OutScaling=2^0
  Integrator : Integrator  InitialConditionSource=external  InitialCondition=0.262753e-3
  Product : Product  OutDataType=sfix(16)  OutScaling=2^0  RndMeth=Zero
  Product1 : Product  OutDataType=sfix(16)  OutScaling=2^0  RndMeth=Zero
  Subtract : Sum  Inputs=+-  OutDataType=sfix(16)  OutScaling=2^-10
  Subtract1 : Sum  Inputs=+-  OutDataType=sfix(16)  OutScaling=2^-10
  nKs : Constant  Value=nKs  OutDataType=sfix(16)  OutScaling=2^0
  tag scope: nKs=global
  wires:
  Product/1 -> Subtract1/2
  Product1/1 -> Subtract1/1
  [alphan] -> Product1/2
  Subtract/1 -> Product1/1
  [betan] -> Product/1
  Integrator/1 -> Product/2, Subtract/2, [nKs]
  Constant/1 -> Subtract/1
  Subtract1/1 -> Integrator/1
  nKs/1 -> Integrator/2

== system Rasmusson/Ionic currents/IKss/aKss ==
  Divide : Product  Inputs=*/  OutDataType=sfix(16)  OutScaling=2^-10
  Integrator : Integrator  InitialConditionSource=external  InitialCondition=0.417069e-3
  Subtract : Sum  Inputs=+-  OutDataType=sfix(16)  OutScaling=2^-10
  aKss : Constant  Value=aKss  OutDataType=sfix(16)  OutScaling=2^0
  tag scope: aKss=global
  wires:
  Integrator/1 -> [aKss], Subtract/2
  Divide/1 -> Integrator/1
  [ass] -> Subtract/1
  [tauKss] -> Divide/2
  Subtract/1 -> Divide/1
  aKss/1 -> Integrator/2

== system Rasmusson/Ionic currents/IKss/iKss ==
  Constant : Constant  Value=0  OutDataType=sfix(16)  OutScaling=2^0
  Integrator : Integrator  InitialConditionSource=external  InitialCondition=1
  iKss : Constant  Value=iKss  OutDataType=sfix(16)  OutScaling=2^0
  tag scope: iKss=global
  wires:
  Constant/1 -> Integrator/1
  Integrator/1 -> [iKss]
  iKss/1 -> Integrator/2

== system Rasmusson/Ionic currents/IKss/tauKss ==
  tauKss : Fcn  Expr=39.3*exp(-0.0862*u)+13.17
  tag scope: tauKss=global
  wires:
  [volt] -> tauKss/1
  tauKss/1 -> [tauKss]

== system Rasmusson/Ionic currents/IKto,f/alphaa ==
  alphaa : Fcn  Expr=0.18064*exp(0.03577*(u+30))
  tag scope: alphaa=global
  wires:
  alphaa/1 -> [alphaa]
  [volt] -> alphaa/1

== system Rasmusson/Ionic currents/IKto,f/alphaj ==
  alphj : Fcn  Expr=(0.000152*exp(-(u+13.5)/7))/(0.067083*exp(-(u+33.5)/7)+1)
  tag scope: alphaj=global
  wires:
  alphj/1 -> [alphaj]
  [volt] -> alphj/1

== system Rasmusson/Ionic currents/IKto,f/atof ==
  Constant : Constant  OutDataType=sfix(16)  OutScaling=2^0
  Integrator : Integrator  InitialConditionSource=external  InitialCondition=0.265563e-2
  Product : Product  OutDataType=sfix(16)  OutScaling=2^0  RndMeth=Zero
  Product1 : Product  OutDataType=sfix(16)  OutScaling=2^0  RndMeth=Zero
  Subtract : Sum  Inputs=+-  OutDataType=sfix(16)  OutScaling=2^-10
  Subtract1 : Sum  Inputs=+-  OutDataType=sfix(16)  OutScaling=2^-10
  ato_f : Constant  Value=ato_f  OutDataType=sfix(16)  OutScaling=2^0
  tag scope: atof=global
  wires:
  Subtract1/1 -> Integrator/1
  Constant/1 -> Subtract/1
  Integrator/1 -> [atof], Subtract/2, Product/2
  [betaa] -> Product/1
  Subtract/1 -> Product1/1
  [alphaa] -> Product1/2
  Product1/1 -> Subtract1/1
  Product/1 -> Subtract1/2
  ato_f/1 -> Integrator/2

== system Rasmusson/Ionic currents/IKto,f/betaa ==
  betaa : Fcn  Expr=0.3956*exp(-0.06237*(u+30))
  tag scope: betaa=global
  wires:
  [volt] -> betaa/1
  betaa/1 -> [betaa]

== system Rasmusson/Ionic currents/IKto,f/betaj ==
  betaj : Fcn  Expr=(0.00095*exp((u+33.5)/7))/(0.051335*exp((u+33.5)/7)+1)
  tag scope: betaj=global
  wires:
  betaj/1 -> [betaj]
  [volt] -> betaj/1

== system Rasmusson/Ionic currents/IKto,f/itof ==
  Constant : Constant  OutDataType=sfix(16)  OutScaling=2^0
  Integrator : Integrator  InitialConditionSource=external  InitialCondition=0.999977
  Product : Product  OutDataType=sfix(16)  OutScaling=2^0  RndMeth=Zero
  Product1 : Product  OutDataType=sfix(16)  OutScaling=2^0  RndMeth=Zero
  Subtract : Sum  Inputs=+-  OutDataType=sfix(16)  OutScaling=2^-10
  Subtract1 : Sum  Inputs=+-  OutDataType=sfix(16)  OutScaling=2^-10
  ito_f : Constant  Value=ito_f  OutDataType=sfix(16)  OutScaling=2^0
  tag scope: itof=global
  wires:
  Integrator/1 -> [itof], Subtract/2, Product1/2
  Subtract1/1 -> Integrator/1
  Product/1 -> Subtract1/1
  Product1/1 -> Subtract1/2
  Subtract/1 -> Product/1
  [alphaj] -> Product/2
  Constant/1 -> Subtract/1
  [betaj] -> Product1/1
  ito_f/1 -> Integrator/2

== system Rasmusson/Ionic currents/IKto,s/ass ==
  ass : Fcn  Expr=1/(1+exp(-(u+22.5)/7.7))
  tag scope: ass=global
  wires:
  [volt] -> ass/1
  ass/1 -> [ass]

== system Rasmusson/Ionic currents/IKto,s/atos ==
  Divide : Product  Inputs=*/  OutDataType=sfix(16)  OutScaling=2^-10
  Integrator : Integrator  InitialConditionSource=external  InitialCondition=0.417069e-3
  Subtract : Sum  Inputs=+-  OutDataType=sfix(16)  OutScaling=2^-10
  ato_s : Constant  Value=ato_s  OutDataType=sfix(16)  OutScaling=2^0
  tag scope: atos=global
  wires:
  Integrator/1 -> [atos], Subtract/2
  Divide/1 -> Integrator/1
  [ass] -> Subtract/1
  [tautas] -> Divide/2
  Subtract/1 -> Divide/1
  ato_s/1 -> Integrator/2

== system Rasmusson/Ionic currents/IKto,s/iss ==
  iss : Fcn  Expr=1/(1+exp((u+45.2)/5.7))
  tag scope: iss=global
  wires:
  iss/1 -> [iss]
  [volt] -> iss/1

== system Rasmusson/Ionic currents/IKto,s/itos ==
  Divide : Product  Inputs=*/  OutDataType=sfix(16)  OutScaling=2^-10
  Integrator : Integrator  InitialConditionSource=external  InitialCondition=0.998543
  Subtract : Sum  Inputs=+-  OutDataType=sfix(16)  OutScaling=2^-10
  ito_s : Constant  Value=ito_s  OutDataType=sfix(16)  OutScaling=2^0
  tag scope: itos=global
  wires:
  Subtract/1 -> Divide/1
  [tautis] -> Divide/2
  [iss] -> Subtract/1
  Divide/1 -> Integrator/1
  Integrator/1 -> Subtract/2, [itos]
  ito_s/1 -> Integrator/2

== system Rasmusson/Ionic currents/IKto,s/tautas ==
  tautas : Fcn  Expr=0.493*exp(-0.0629*u)+2.058
  tag scope: tautas=global
  wires:
  [volt] -> tautas/1
  tautas/1 -> [tautas]

== system Rasmusson/Ionic currents/IKto,s/tautis ==
  tautis : Fcn  Expr=270+1050/(1+exp((u+45.2)/5.7))
  tag scope: tautis=global
  wires:
  tautis/1 -> [tautis]
  [volt] -> tautis/1

== system Rasmusson/Ionic currents/IKur/aur ==
  Divide : Product  Inputs=*/  OutDataType=sfix(16)  OutScaling=2^-10
  Integrator : Integrator  InitialConditionSource=external  InitialCondition=0.417069e-3
  Subtract : Sum  Inputs=+-  OutDataType=sfix(16)  OutScaling=2^-10
  aur : Constant  Value=aur  OutDataType=sfix(16)  OutScaling=2^0
  tag scope: aur=global
  wires:
  Subtract/1 -> Divide/1
  [tauaur] -> Divide/2
  [ass] -> Subtract/1
  Divide/1 -> Integrator/1
  Integrator/1 -> Subtract/2, [aur]
  aur/1 -> Integrator/2

== system Rasmusson/Ionic currents/IKur/iur ==
  Divide : Product  Inputs=*/  OutDataType=sfix(16)  OutScaling=2^-10
  Integrator : Integrator  InitialConditionSource=external  InitialCondition=0.998543
  Subtract : Sum  Inputs=+-  OutDataType=sfix(16)  OutScaling=2^-10
  iur : Constant  Value=iur  OutDataType=sfix(16)  OutScaling=2^0
  tag scope: iur=global
  wires:
  Integrator/1 -> [iur], Subtract/2
  Divide/1 -> Integrator/1
  [iss] -> Subtract/1
  [tauiur] -> Divide/2
  Subtract/1 -> Divide/1
  iur/1 -> Integrator/2

== system Rasmusson/Ionic currents/IKur/tauaur ==
  tauaur : Fcn  Expr=0.493*exp(-0.0629*u)+2.058
  tag scope: tauaur=global
  wires:
  tauaur/1 -> [tauaur]
  [volt] -> tauaur/1

== system Rasmusson/Ionic currents/IKur/tauiur ==
  tauiur : Fcn  Expr=1200-170/(1+exp((u+45.2)/5.7))
  tag scope: tauiur=global
  wires:
  [volt] -> tauiur/1
  tauiur/1 -> [tauiur]

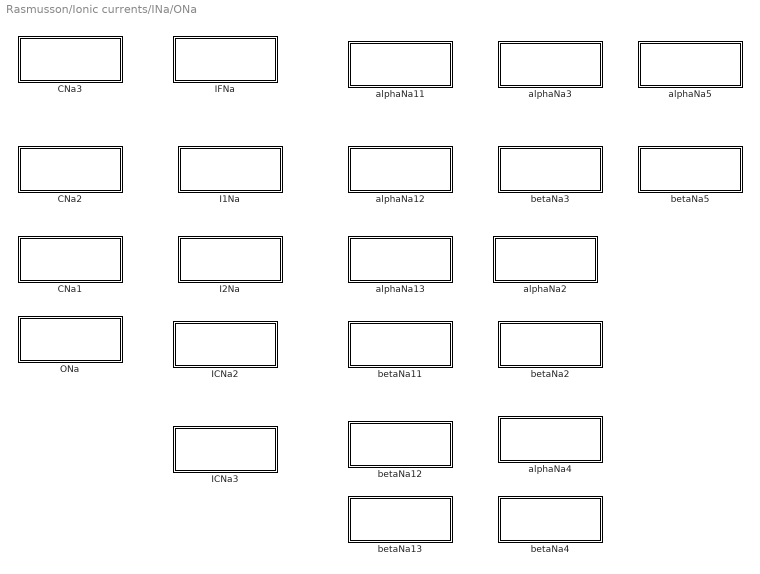
== system Rasmusson/Ionic currents/INa/ONa ==
  CNa1 : Subsystem
  CNa2 : Subsystem
  CNa3 : Subsystem
  I1Na : Subsystem
  I2Na : Subsystem
  ICNa2 : Subsystem
  ICNa3 : Subsystem
  IFNa : Subsystem
  ONa : Subsystem
  alphaNa11 : Subsystem
  alphaNa12 : Subsystem
  alphaNa13 : Subsystem
  alphaNa2 : Subsystem
  alphaNa3 : Subsystem
  alphaNa4 : Subsystem
  alphaNa5 : Subsystem
  betaNa11 : Subsystem
  betaNa12 : Subsystem
  betaNa13 : Subsystem
  betaNa2 : Subsystem
  betaNa3 : Subsystem
  betaNa4 : Subsystem
  betaNa5 : Subsystem

== system Rasmusson/Ionic currents/INaK/fNaK ==
  Add : Sum  Inputs=+++  OutDataType=sfix(16)  OutScaling=2^-10
  Constant : Constant  OutDataType=sfix(16)  OutScaling=2^0
  Fcn : Fcn  Expr=1/u
  Gain : Gain  Gain=0.1245  ParameterDataType=sfix(16)  ParameterScaling=2^0  OutDataType=sfix(16)  OutScaling=2^0
  Gain1 : Gain  Gain=-0.1  ParameterDataType=sfix(16)  ParameterScaling=2^0  OutDataType=sfix(16)  OutScaling=2^0
  Gain2 : Gain  Gain=0.0365  ParameterDataType=sfix(16)  ParameterScaling=2^0  OutDataType=sfix(16)  OutScaling=2^0
  Gain3 : Gain  Gain=-1  ParameterDataType=sfix(16)  ParameterScaling=2^0  OutDataType=sfix(16)  OutScaling=2^0
  Math Function : Math  OutDataType=sfix(16)  OutScaling=2^0  SaturateOnIntegerOverflow=on
  Math Function1 : Math  OutDataType=sfix(16)  OutScaling=2^0  SaturateOnIntegerOverflow=on
  Product : Product  OutDataType=sfix(16)  OutScaling=2^0  RndMeth=Zero
  sigma : Subsystem
  tag scope: fNaK=global
  wires:
  Fcn/1 -> [fNaK]
  Add/1 -> Fcn/1
  Constant/1 -> Add/1
  Gain/1 -> Add/2
  Math Function/1 -> Gain/1
  Gain1/1 -> Math Function/1
  [VFdivideRT] -> Gain1/1, Gain3/1
  Gain2/1 -> Add/3
  Product/1 -> Gain2/1
  Math Function1/1 -> Product/2
  Gain3/1 -> Math Function1/1
  [sigma] -> Product/1

== system Rasmusson/Voltage/ICaCl/OClCa ==
  OClCa : Fcn  Expr=0.2/(1+exp(-(u-46.7)/7.8))
  tag scope: OClCa=global
  wires:
  [volt] -> OClCa/1
  OClCa/1 -> [OClCa]

== system Rasmusson/Concentrations/Caconcentration/Cabuffering/HTRPNCa ==
  HTRPNCa : Constant  Value=HTRPNCa  OutDataType=sfix(16)  OutScaling=2^0
  HTRPNtot : Constant  Value=HTRPN_tot  OutDataType=sfix(16)  OutScaling=2^0
  Integrator : Integrator  InitialConditionSource=external  InitialCondition=125.29
  Product : Product  Inputs=3  OutDataType=sfix(16)  OutScaling=2^0  RndMeth=Zero
  Product1 : Product  OutDataType=sfix(16)  OutScaling=2^0  RndMeth=Zero
  Subtract : Sum  Inputs=+-  OutDataType=sfix(16)  OutScaling=2^-10
  Subtract1 : Sum  Inputs=+-  OutDataType=sfix(16)  OutScaling=2^-10
  khtrpn+ : Constant  Value=khtrpn1  OutDataType=sfix(16)  OutScaling=2^0
  khtrpn- : Constant  Value=khtrpn2  OutDataType=sfix(16)  OutScaling=2^0
  tag scope: HTRPNCa=global
  wires:
  khtrpn-/1 -> Product1/1
  HTRPNtot/1 -> Subtract1/1
  Subtract1/1 -> Product/3
  [Cai] -> Product/2
  khtrpn+/1 -> Product/1
  Product1/1 -> Subtract/2
  Product/1 -> Subtract/1
  Subtract/1 -> Integrator/1
  Integrator/1 -> Product1/2, Subtract1/2, [HTRPNCa]
  HTRPNCa/1 -> Integrator/2

== system Rasmusson/Concentrations/Caconcentration/Cabuffering/LTRPNCa ==
  Integrator : Integrator  InitialConditionSource=external  InitialCondition=11.2684
  LTRPNCa : Constant  Value=LTRPNCa  OutDataType=sfix(16)  OutScaling=2^0
  LTRPNtot : Constant  Value=LTRPN_tot  OutDataType=sfix(16)  OutScaling=2^0
  Product : Product  Inputs=3  OutDataType=sfix(16)  OutScaling=2^0  RndMeth=Zero
  Product1 : Product  OutDataType=sfix(16)  OutScaling=2^0  RndMeth=Zero
  Subtract : Sum  Inputs=+-  OutDataType=sfix(16)  OutScaling=2^-10
  Subtract1 : Sum  Inputs=+-  OutDataType=sfix(16)  OutScaling=2^-10
  kltrpn+ : Constant  Value=kltrpn1  OutDataType=sfix(16)  OutScaling=2^0
  kltrpn- : Constant  Value=kltrpn2  OutDataType=sfix(16)  OutScaling=2^0
  tag scope: LTRPNCa=global
  wires:
  Integrator/1 -> [LTRPNCa], Subtract1/2, Product1/2
  Subtract/1 -> Integrator/1
  Product/1 -> Subtract/1
  Product1/1 -> Subtract/2
  kltrpn+/1 -> Product/1
  [Cai] -> Product/2
  Subtract1/1 -> Product/3
  LTRPNtot/1 -> Subtract1/1
  kltrpn-/1 -> Product1/1
  LTRPNCa/1 -> Integrator/2

== system Rasmusson/Concentrations/Caconcentration/Caconcentration/BJSR ==
  Add : Sum  OutDataType=sfix(16)  OutScaling=2^-10
  Add1 : Sum  OutDataType=sfix(16)  OutScaling=2^-10
  CSQNtot : Constant  Value=CSQN_tot  OutDataType=sfix(16)  OutScaling=2^0
  Constant : Constant  OutDataType=sfix(16)  OutScaling=2^0
  Divide : Product  Inputs=**/  OutDataType=sfix(16)  OutScaling=2^-10
  Fcn : Fcn  Expr=1/u
  KmCSQN : Constant  Value=Km_CSQN  OutDataType=sfix(16)  OutScaling=2^0
  Math Function : Math  Operator=square  OutDataType=sfix(16)  OutScaling=2^0  SaturateOnIntegerOverflow=on
  tag scope: BJSR=global
  wires:
  Fcn/1 -> [BJSR]
  Add/1 -> Fcn/1
  Constant/1 -> Add/1
  Divide/1 -> Add/2
  CSQNtot/1 -> Divide/1
  KmCSQN/1 -> Divide/2, Add1/1
  Math Function/1 -> Divide/3
  Add1/1 -> Math Function/1
  [CaJSR] -> Add1/2

== system Rasmusson/Concentrations/Caconcentration/Caconcentration/Bi ==
  Add : Sum  OutDataType=sfix(16)  OutScaling=2^-10
  Add1 : Sum  OutDataType=sfix(16)  OutScaling=2^-10
  CMDNtot : Constant  Value=CMDN_tot  OutDataType=sfix(16)  OutScaling=2^0
  Constant : Constant  OutDataType=sfix(16)  OutScaling=2^0
  Divide : Product  Inputs=**/  OutDataType=sfix(16)  OutScaling=2^-10
  Fcn : Fcn  Expr=1/u
  KmCMDN : Constant  Value=Km_CMDN  OutDataType=sfix(16)  OutScaling=2^0
  Math Function : Math  Operator=square  OutDataType=sfix(16)  OutScaling=2^0  SaturateOnIntegerOverflow=on
  tag scope: Bi=global
  wires:
  Fcn/1 -> [Bi]
  Add/1 -> Fcn/1
  Constant/1 -> Add/1
  Divide/1 -> Add/2
  CMDNtot/1 -> Divide/1
  KmCMDN/1 -> Divide/2, Add1/1
  Math Function/1 -> Divide/3
  Add1/1 -> Math Function/1
  [Cai] -> Add1/2

== system Rasmusson/Concentrations/Caconcentration/Caconcentration/Bss ==
  Add : Sum  OutDataType=sfix(16)  OutScaling=2^-10
  Add1 : Sum  OutDataType=sfix(16)  OutScaling=2^-10
  CMDNtot : Constant  Value=CMDN_tot  OutDataType=sfix(16)  OutScaling=2^0
  Constant : Constant  OutDataType=sfix(16)  OutScaling=2^0
  Divide : Product  Inputs=**/  OutDataType=sfix(16)  OutScaling=2^-10
  Fcn : Fcn  Expr=1/u
  KmCMDN : Constant  Value=Km_CMDN  OutDataType=sfix(16)  OutScaling=2^0
  Math Function : Math  Operator=square  OutDataType=sfix(16)  OutScaling=2^0  SaturateOnIntegerOverflow=on
  tag scope: Bss=global
  wires:
  [Cass] -> Add1/2
  Add1/1 -> Math Function/1
  Math Function/1 -> Divide/3
  KmCMDN/1 -> Add1/1, Divide/2
  CMDNtot/1 -> Divide/1
  Divide/1 -> Add/2
  Constant/1 -> Add/1
  Add/1 -> Fcn/1
  Fcn/1 -> [Bss]

== system Rasmusson/Concentrations/Caconcentration/Caconcentration/CaJSR ==
  CaJSR : Constant  Value=CaJSR  OutDataType=sfix(16)  OutScaling=2^0
  Integrator : Integrator  InitialConditionSource=external  InitialCondition=1299.5
  Product : Product  OutDataType=sfix(16)  OutScaling=2^0  RndMeth=Zero
  Subtract : Sum  Inputs=+-  OutDataType=sfix(16)  OutScaling=2^-10
  tag scope: CaJSR=global
  wires:
  Integrator/1 -> [CaJSR]
  Product/1 -> Integrator/1
  [BJSR] -> Product/1
  Subtract/1 -> Product/2
  [Jtr] -> Subtract/1
  [Jrel] -> Subtract/2
  CaJSR/1 -> Integrator/2

== system Rasmusson/Concentrations/Caconcentration/Caconcentration/CaNSR ==
  Constant : Constant  Value=CaNSR  OutDataType=sfix(16)  OutScaling=2^0
  Divide : Product  Inputs=**/  OutDataType=sfix(16)  OutScaling=2^-10
  Divide2 : Product  Inputs=**/  OutDataType=sfix(16)  OutScaling=2^-10
  Integrator : Integrator  InitialConditionSource=external  InitialCondition=1299.5
  Subtract : Sum  Inputs=+-  OutDataType=sfix(16)  OutScaling=2^-10
  Subtract1 : Sum  Inputs=+-  OutDataType=sfix(16)  OutScaling=2^-10
  VJSR : Constant  Value=VJSR  OutDataType=sfix(16)  OutScaling=2^0
  VNSR : Constant  Value=VNSR  OutDataType=sfix(16)  OutScaling=2^0
  Vmyo : Constant  Value=Vmyo  OutDataType=sfix(16)  OutScaling=2^0
  tag scope: CaNSR=global
  wires:
  [Jleak] -> Subtract/2
  [Jup] -> Subtract/1
  Vmyo/1 -> Divide/1
  Integrator/1 -> [CaNSR]
  Subtract1/1 -> Integrator/1
  Divide/1 -> Subtract1/1
  Divide2/1 -> Subtract1/2
  Subtract/1 -> Divide/2
  VNSR/1 -> Divide/3, Divide2/3
  VJSR/1 -> Divide2/1
  [Jtr] -> Divide2/2
  Constant/1 -> Integrator/2
